simulink model "sim_sistema_1"  (Simulink 9.0)
settings: Solver=ode3  StartTime=0.0  StopTime=5  FixedStep=1e-4  RelTol=1e-3  EnableMultiTasking=on
values from neighbouring files (symbols this model uses):
  A = [0 1 0 ... (first row only)    [sistema_1.m]
  B = [0;0;1]    [sistema_1.m]
  C = eye(3)    [sistema_1.m]
  D = [0;0;0]    [sistema_1.m]
  K = acker(A,B,s)    [sistema_1.m]
settings Model: Creator=taniel.franklin  LastModifiedBy=taniel.franklin
settings DataIOCC: LimitDataPoints=on  SignalLoggingSaveFormat=ModelDataLogs
settings OptimizationCC: ExpressionDepthLimit=2147483647
settings DebuggingCC: SolverPrmCheckMsg=warning  FcnCallInpInsideContextMsg=warning  StateNameClashWarn=warning
settings GRTTargetCC: GeneratePreprocessorConditionals=Disable all  CombineOutputUpdateFcns=off  GRTInterface=on

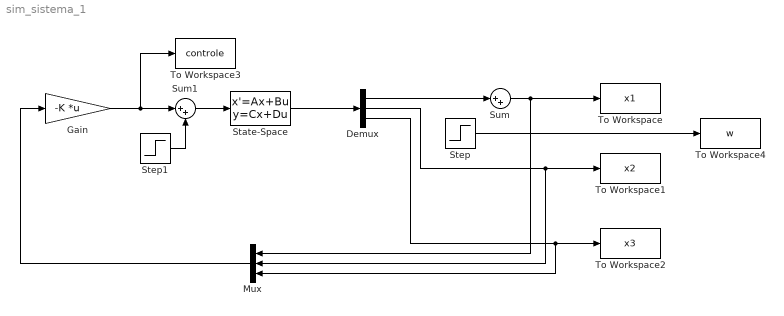
== system sim_sistema_1 ==
  Demux : Demux  Outputs=3
  Gain : Gain  Gain=-K  Multiplication=Matrix(K*u)
  Mux : Mux  Inputs=3
  State-Space : StateSpace  A=A  B=B  C=C  D=D  InitialCondition=[0;0;0]
  Step : Step  Time=0.5  SampleTime=0
  Step1 : Step  SampleTime=0
  Sum : Sum  Inputs=|++
  Sum1 : Sum  Inputs=|++
  To Workspace : ToWorkspace  VariableName=x1  SaveFormat=Structure With Time  SampleTime=-1
  To Workspace1 : ToWorkspace  VariableName=x2  SaveFormat=Structure With Time  SampleTime=-1
  To Workspace2 : ToWorkspace  VariableName=x3  SaveFormat=Structure With Time  SampleTime=-1
  To Workspace3 : ToWorkspace  VariableName=controle  SaveFormat=Structure With Time  SampleTime=-1
  To Workspace4 : ToWorkspace  VariableName=w  SaveFormat=Structure With Time  SampleTime=-1
  wires:
  State-Space/1 -> Demux/1
  Demux/2 -> To Workspace1/1, Mux/2
  Demux/3 -> To Workspace2/1, Mux/3
  Gain/1 -> Sum1/1, To Workspace3/1
  Sum/1 -> To Workspace/1, Mux/1
  Demux/1 -> Sum/1
  Step/1 -> To Workspace4/1
  Mux/1 -> Gain/1
  Sum1/1 -> State-Space/1
  Step1/1 -> Sum1/2
